simulink model "untitled"  (R2019a)
settings: Solver=VariableStepAuto  StartTime=0.0  StopTime=4  RelTol=1e-3
libraries: Department x1
settings Model: Creator=arsineh  LastModifiedBy=arsineh

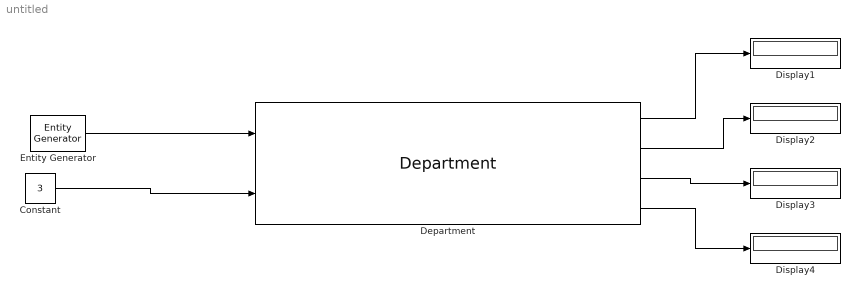
== system untitled ==
  Constant : Constant  Value=3
  Department : Department/Department  SystemSampleTime=-1
  Display{1..4} (4 alike) : Display
  Entity Generator : EntityGenerator  OutputPortMessageModes=m  EntityType=Structured  EntityTypeName=Entity
  wires:
  Entity Generator/1 -> Department/1
  Constant/1 -> Department/2
  Department/1 -> Display1/1
  Department/2 -> Display2/1
  Department/3 -> Display3/1
  Department/4 -> Display4/1
